simulink model "fft_wideband_real"  (R2012b)
settings: Solver=ode45  StartTime=0.0  StopTime=19999  RelTol=1e-3
undefined symbols (not defined in the file): fft_wideband_real_shift_schedule_user_data_out
libraries: xbsIndex_r4 x8703, xbsReplacements_r4 x36, xps_library x24, dspsigops x16, simulink_xsg_bridge x1
(part 8 of 51)

== system fft_wideband_real/fft_wideband_real/phase_mult/phase12_coeffs ==
  rst : Inport
  Counter : xbsIndex_r4/Counter  cnt_type=Free Running  cnt_to=Inf  operation=Up  start_count=0  cnt_by_val=1  arith_type=Unsigned  n_bits=6  bin_pt=0  load_pin=off  rst=on  en=off  explicit_period=on  period=1  dbl_ovrd=off  use_behavioral_HDL=off  implementation=Fabric  block_type=counter
  Slice : xbsIndex_r4/Slice  nbits=6  boolean_output=off  mode=Upper Bit Location + Width  bit1=0  base1=MSB of Input  bit0=0  base0=LSB of Input  dbl_ovrd=off  block_type=slice
  bram_din_const : xbsIndex_r4/Constant  const=0  gui_display_data_type=Fixed-point  arith_type=Signed (2's comp)  n_bits=18  bin_pt=17  preci_type=Single  exp_width=8  frac_width=24  explicit_period=off  period=1  equ=P=C  opselect=C  inp2=PCIN>>17  opr=+  inp1=P  carry=CIN  dbl_ovrd=off  block_type=constant
  bram_we_const : xbsIndex_r4/Constant  const=0  gui_display_data_type=Fixed-point  arith_type=Boolean  n_bits=16  bin_pt=14  preci_type=Single  exp_width=8  frac_width=24  explicit_period=off  period=1  equ=P=C  opselect=C  inp2=PCIN>>17  opr=+  inp1=P  carry=CIN  dbl_ovrd=off  block_type=constant
  cnt_sign_exta : xbsIndex_r4/Convert  gui_display_data_type=Fixed-point  arith_type=Unsigned  n_bits=10  bin_pt=0  float_type=Single  exp_bits=8  fraction_bits=24  quantization=Truncate  overflow=Wrap  en=off  latency=0  dbl_ovrd=off  pipeline=off  block_type=convert
  cnt_sign_extb : xbsIndex_r4/Convert  gui_display_data_type=Fixed-point  arith_type=Unsigned  n_bits=9  bin_pt=0  float_type=Single  exp_bits=8  fraction_bits=24  quantization=Truncate  overflow=Wrap  en=off  latency=0  dbl_ovrd=off  pipeline=off  block_type=convert
  coeff_mem : xbsIndex_r4/Dual Port RAM  depth=1024  initVector=[1 0.997726440429688 0.99090576171875 0.979568481445312 0.963775634765625 0.943595886230469 0.919113159179688 0.890449523925781 0.85772705078125 0.82110595703125 0.780738830566406 0.73681640625 0.689537048339844 0.639122009277344 0.585800170898438 0.529800415039062 0.471397399902344 0.410842895507812 0.348419189453125 0.284408569335938 0.219100952148438 0.152793884277344 0.0858001708984375 0.0184097290039062 -0.0490646362304688 -0.116317749023438 -0.183036804199219 -0.248924255371094 -0.313682556152344 -0.377006530761719 -0.438613891601562 -0.49822998046875 -0.555572509765625 -0.610382080078125 -0.66241455078125 -0.711433410644531 -0.757209777832031 -0.799537658691406 -0.838226318359375 -0.873092651367188 -0.90399169921875 -0.930763244628906 -0.95330810546875 -0.971504211425781 -0.985275268554688 -0.99456787109375 -0.999320983886719 -0.999526977539062 -0.995185852050781 -0.986305236816406 -0.972938537597656 -0.95513916015625 -0.932991027832031 -0.906593322753906 -0.876068115234375 -0.841552734375 -0.803207397460938 -0.761199951171875 -0.715728759765625 -0.666999816894531 -0.615234375 -0.560661315917969 -0.5035400390625 -0.444122314453125 0 0 0 0 0 0 0 0 0 0 0 0 0 0 0 0 0 0 0 0 0 0 0 0 0 0 0 0 0 0 0 0 0 0 0 0 0 0 0 0 0 0 0 0 0 0 0 0 0 0 0 0 0 0 0 0 0 0 0 0 0 0 0 0 0 0 0 0 0 0 0 0 0 0 0 0 0 0 0 0 0 0 0 0 0 0 0 0 0 0 0 0 0 0 0 0 0 0 0 0 0 0 0 0 0 0 0 0 0 0 0 0 0 0 0 0 0 0 0 0 0 0 0 0 0 0 0 0 0 0 0 0 0 0 0 0 0 0 0 0 0 0 0 0 0 0 0 0 0 0 0 0 0 0 0 0 0 0 0 0 0 0 0 0 0 0 0 0 0 0 0 0 0 0 0 0 0 0 0 0 0 0 0 0 0 0 0 0 0 0 0 0 0 0 0 0 0 0 0 0 0 0 0 0 0 0 0 0 0 0 0 0 0 0 0 0 0 0 0 0 0 0 0 0 0 0 0 0 0 0 0 0 0 0 0 0 0 0 0 0 0 0 0 0 0 0 0 0 0 0 0 0 0 0 0 0 0 0 0 0 0 0 0 0 0 0 0 0 0 0 0 0 0 0 0 0 0 0 0 0 0 0 0 0 0 0 0 0 0 0 0 0 0 0 0 0 0 0 0 0 0 0 0 0 0 0 0 0 0 0 0 0 0 0 0 0 0 0 0 0 0 0 0 0 0 0 0 0 0 0 0 0 0 0 0 0 0 0 0 0 0 0 0 0 0 0 0 0 0 0 0 0 0 0 0 0 0 0 0 0 0 0 0 0 0 0 0 0 0 0 0 0 0 0 0 0 0 0 0 0 0 0 0 0 0 0 0 0 0 0 0 0 0 0 0 0 0 0 0 0 0 0 0 0 0 0 0 0 0 0 0 0 0 0 0 0 0 0 0 0 0 0 0 0 0 0 0 0 0 0 0 0 0 0 0 0 0 0 0 0 0 0 0 0 0 0 0 0 0 -0.06744384765625 -0.13458251953125 -0.201103210449219 -0.266716003417969 -0.331108093261719 -0.393989562988281 -0.455085754394531 -0.51409912109375 -0.570777893066406 -0.624862670898438 -0.676094055175781 -0.724250793457031 -0.76910400390625 -0.810455322265625 -0.848121643066406 -0.881919860839844 -0.911705017089844 -0.937339782714844 -0.958702087402344 -0.975700378417969 -0.988258361816406 -0.996315002441406 -0.999832153320312 -0.998794555664062 -0.993209838867188 -0.983108520507812 -0.968521118164062 -0.949531555175781 -0.92620849609375 -0.898674011230469 -0.867042541503906 -0.831466674804688 -0.792106628417969 -0.749137878417969 -0.702751159667969 -0.653175354003906 -0.600616455078125 -0.545326232910156 -0.487548828125 -0.427558898925781 -0.365615844726562 -0.302009582519531 -0.237022399902344 -0.17095947265625 -0.104118347167969 -0.03680419921875 0.0306777954101562 0.0980148315429688 0.164909362792969 0.231056213378906 0.296150207519531 0.359893798828125 0.4219970703125 0.482185363769531 0.540168762207031 0.595695495605469 0.648513793945312 0.698379516601562 0.74505615234375 0.788345336914062 0.828048706054688 0.863975524902344 0.895965576171875 0 0 0 0 0 0 0 0 0 0 0 0 0 0 0 0 0 0 0 0 0 0 0 0 0 0 0 0 0 0 0 0 0 0 0 0 0 0 0 0 0 0 0 0 0 0 0 0 0 0 0 0 0 0 0 0 0 0 0 0 0 0 0 0 0 0 0 0 0 0 0 0 0 0 0 0 0 0 0 0 0 0 0 0 0 0 0 0 0 0 0 0 0 0 0 0 0 0 0 0 0 0 0 0 0 0 0 0 0 0 0 0 0 0 0 0 0 0 0 0 0 0 0 0 0 0 0 0 0 0 0 0 0 0 0 0 0 0 0 0 0 0 0 0 0 0 0 0 0 0 0 0 0 0 0 0 0 0 0 0 0 0 0 0 0 0 0 0 0 0 0 0 0 0 0 0 0 0 0 0 0 0 0 0 0 0 0 0 0 0 0 0 0 0 0 0 0 0 0 0 0 0 0 0 0 0 0 0 0 0 0 0 0 0 0 0 0 0 0 0 0 0 0 0 0 0 0 0 0 0 0 0 0 0 0 0 0 0 0 0 0 0 0 0 0 0 0 0 0 0 0 0 0 0 0 0 0 0 0 0 0 0 0 0 0 0 0 0 0 0 0 0 0 0 0 0 0 0 0 0 0 0 0 0 0 0 0 0 0 0 0 0 0 0 0 0 0 0 0 0 0 0 0 0 0 0 0 0 0 0 0 0 0 0 0 0 0 0 0 0 0 0 0 0 0 0 0 0 0 0 0 0 0 0 0 0 0 0 0 0 0 0 0 0 0 0 0 0 0 0 0 0 0 0 0 0 0 0 0 0 0 0 0 0 0 0 0 0 0 0 0 0 0 0 0 0 0 0 0 0 0 0 0 0 0 0 0 0 0 0 0 0 0 0 0 0 0 0 0 0 0 0 0 0 0 0 0 0 0 0 0 0 0 0 0 0 0 0 0 0 0 0 0 0 0 0 0 0 0 0 0 0 0 0 0 0 0 0 0 0 0 0 0 0 0 0 0 0]  distributed_mem=Block RAM  init_a=0  init_b=0  rst_a=off  rst_b=off  en_a=off  en_b=off  latency=2  write_mode_A=Read After Write  write_mode_B=Read After Write  dbl_ovrd=off  optimize=Area  use_rpm=on  block_type=dpram
  counter_b_concat : xbsIndex_r4/Concat  num_inputs=2  dbl_ovrd=off  block_type=concat
  counter_b_pad : xbsIndex_r4/Constant  const=1  gui_display_data_type=Fixed-point  arith_type=Unsigned  n_bits=1  bin_pt=0  preci_type=Single  exp_width=8  frac_width=24  explicit_period=off  period=1  equ=P=C  opselect=C  inp2=PCIN>>17  opr=+  inp1=P  carry=CIN  dbl_ovrd=off  block_type=constant
  ri_to_c : Subsystem
  w : Outport
  wires:
  Slice/1 -> cnt_sign_extb/1, cnt_sign_exta/1
  bram_din_const/1 -> coeff_mem/5, coeff_mem/2
  bram_we_const/1 -> coeff_mem/6, coeff_mem/3
  ri_to_c/1(c) -> w/1
  coeff_mem/2 -> ri_to_c/2(im)
  coeff_mem/1 -> ri_to_c/1(re)
  counter_b_concat/1 -> coeff_mem/4
  cnt_sign_exta/1 -> coeff_mem/1
  cnt_sign_extb/1 -> counter_b_concat/2
  counter_b_pad/1 -> counter_b_concat/1
  Counter/1 -> Slice/1
  rst/1 -> Counter/1

== system fft_wideband_real/fft_wideband_real/phase_mult/phase13_coeffs ==
  rst : Inport
  Counter : xbsIndex_r4/Counter  cnt_type=Free Running  cnt_to=Inf  operation=Up  start_count=0  cnt_by_val=1  arith_type=Unsigned  n_bits=6  bin_pt=0  load_pin=off  rst=on  en=off  explicit_period=on  period=1  dbl_ovrd=off  use_behavioral_HDL=off  implementation=Fabric  block_type=counter
  Slice : xbsIndex_r4/Slice  nbits=6  boolean_output=off  mode=Upper Bit Location + Width  bit1=0  base1=MSB of Input  bit0=0  base0=LSB of Input  dbl_ovrd=off  block_type=slice
  bram_din_const : xbsIndex_r4/Constant  const=0  gui_display_data_type=Fixed-point  arith_type=Signed (2's comp)  n_bits=18  bin_pt=17  preci_type=Single  exp_width=8  frac_width=24  explicit_period=off  period=1  equ=P=C  opselect=C  inp2=PCIN>>17  opr=+  inp1=P  carry=CIN  dbl_ovrd=off  block_type=constant
  bram_we_const : xbsIndex_r4/Constant  const=0  gui_display_data_type=Fixed-point  arith_type=Boolean  n_bits=16  bin_pt=14  preci_type=Single  exp_width=8  frac_width=24  explicit_period=off  period=1  equ=P=C  opselect=C  inp2=PCIN>>17  opr=+  inp1=P  carry=CIN  dbl_ovrd=off  block_type=constant
  cnt_sign_exta : xbsIndex_r4/Convert  gui_display_data_type=Fixed-point  arith_type=Unsigned  n_bits=10  bin_pt=0  float_type=Single  exp_bits=8  fraction_bits=24  quantization=Truncate  overflow=Wrap  en=off  latency=0  dbl_ovrd=off  pipeline=off  block_type=convert
  cnt_sign_extb : xbsIndex_r4/Convert  gui_display_data_type=Fixed-point  arith_type=Unsigned  n_bits=9  bin_pt=0  float_type=Single  exp_bits=8  fraction_bits=24  quantization=Truncate  overflow=Wrap  en=off  latency=0  dbl_ovrd=off  pipeline=off  block_type=convert
  coeff_mem : xbsIndex_r4/Dual Port RAM  depth=1024  initVector=[1 0.997291564941406 0.989173889160156 0.975700378417969 0.956939697265625 0.932991027832031 0.90399169921875 0.870086669921875 0.831466674804688 0.788345336914062 0.740951538085938 0.689537048339844 0.634391784667969 0.5758056640625 0.51409912109375 0.449607849121094 0.382682800292969 0.313682556152344 0.24298095703125 0.17095947265625 0.0980148315429688 0.0245437622070312 -0.0490646362304688 -0.122413635253906 -0.195091247558594 -0.266716003417969 -0.336891174316406 -0.405242919921875 -0.471397399902344 -0.534996032714844 -0.595695495605469 -0.653175354003906 -0.707107543945312 -0.757209777832031 -0.803207397460938 -0.844856262207031 -0.881919860839844 -0.914207458496094 -0.941543579101562 -0.963775634765625 -0.980781555175781 -0.992477416992188 -0.998794555664062 -0.999702453613281 -0.995185852050781 -0.985275268554688 -0.97003173828125 -0.949531555175781 -0.923881530761719 -0.893226623535156 -0.85772705078125 -0.817581176757812 -0.77301025390625 -0.724250793457031 -0.671562194824219 -0.615234375 -0.555572509765625 -0.492897033691406 -0.427558898925781 -0.359893798828125 -0.290283203125 -0.219100952148438 -0.146728515625 -0.0735626220703125 0 0 0 0 0 0 0 0 0 0 0 0 0 0 0 0 0 0 0 0 0 0 0 0 0 0 0 0 0 0 0 0 0 0 0 0 0 0 0 0 0 0 0 0 0 0 0 0 0 0 0 0 0 0 0 0 0 0 0 0 0 0 0 0 0 0 0 0 0 0 0 0 0 0 0 0 0 0 0 0 0 0 0 0 0 0 0 0 0 0 0 0 0 0 0 0 0 0 0 0 0 0 0 0 0 0 0 0 0 0 0 0 0 0 0 0 0 0 0 0 0 0 0 0 0 0 0 0 0 0 0 0 0 0 0 0 0 0 0 0 0 0 0 0 0 0 0 0 0 0 0 0 0 0 0 0 0 0 0 0 0 0 0 0 0 0 0 0 0 0 0 0 0 0 0 0 0 0 0 0 0 0 0 0 0 0 0 0 0 0 0 0 0 0 0 0 0 0 0 0 0 0 0 0 0 0 0 0 0 0 0 0 0 0 0 0 0 0 0 0 0 0 0 0 0 0 0 0 0 0 0 0 0 0 0 0 0 0 0 0 0 0 0 0 0 0 0 0 0 0 0 0 0 0 0 0 0 0 0 0 0 0 0 0 0 0 0 0 0 0 0 0 0 0 0 0 0 0 0 0 0 0 0 0 0 0 0 0 0 0 0 0 0 0 0 0 0 0 0 0 0 0 0 0 0 0 0 0 0 0 0 0 0 0 0 0 0 0 0 0 0 0 0 0 0 0 0 0 0 0 0 0 0 0 0 0 0 0 0 0 0 0 0 0 0 0 0 0 0 0 0 0 0 0 0 0 0 0 0 0 0 0 0 0 0 0 0 0 0 0 0 0 0 0 0 0 0 0 0 0 0 0 0 0 0 0 0 0 0 0 0 0 0 0 0 0 0 0 0 0 0 0 0 0 0 0 0 0 0 0 0 0 0 0 0 0 0 0 0 0 0 0 0 0 0 0 0 0 0 0 0 0 0 0 0 0 0 0 0 0 0 0 0 0 0 0 0 0 0 -0.0735626220703125 -0.146728515625 -0.219100952148438 -0.290283203125 -0.359893798828125 -0.427558898925781 -0.492897033691406 -0.555572509765625 -0.615234375 -0.671562194824219 -0.724250793457031 -0.77301025390625 -0.817581176757812 -0.85772705078125 -0.893226623535156 -0.923881530761719 -0.949531555175781 -0.97003173828125 -0.985275268554688 -0.995185852050781 -0.999702453613281 -0.998794555664062 -0.992477416992188 -0.980781555175781 -0.963775634765625 -0.941543579101562 -0.914207458496094 -0.881919860839844 -0.844856262207031 -0.803207397460938 -0.757209777832031 -0.707107543945312 -0.653175354003906 -0.595695495605469 -0.534996032714844 -0.471397399902344 -0.405242919921875 -0.336891174316406 -0.266716003417969 -0.195091247558594 -0.122413635253906 -0.0490646362304688 0.0245437622070312 0.0980148315429688 0.17095947265625 0.24298095703125 0.313682556152344 0.382682800292969 0.449607849121094 0.51409912109375 0.5758056640625 0.634391784667969 0.689537048339844 0.740951538085938 0.788345336914062 0.831466674804688 0.870086669921875 0.90399169921875 0.932991027832031 0.956939697265625 0.975700378417969 0.989173889160156 0.997291564941406 0 0 0 0 0 0 0 0 0 0 0 0 0 0 0 0 0 0 0 0 0 0 0 0 0 0 0 0 0 0 0 0 0 0 0 0 0 0 0 0 0 0 0 0 0 0 0 0 0 0 0 0 0 0 0 0 0 0 0 0 0 0 0 0 0 0 0 0 0 0 0 0 0 0 0 0 0 0 0 0 0 0 0 0 0 0 0 0 0 0 0 0 0 0 0 0 0 0 0 0 0 0 0 0 0 0 0 0 0 0 0 0 0 0 0 0 0 0 0 0 0 0 0 0 0 0 0 0 0 0 0 0 0 0 0 0 0 0 0 0 0 0 0 0 0 0 0 0 0 0 0 0 0 0 0 0 0 0 0 0 0 0 0 0 0 0 0 0 0 0 0 0 0 0 0 0 0 0 0 0 0 0 0 0 0 0 0 0 0 0 0 0 0 0 0 0 0 0 0 0 0 0 0 0 0 0 0 0 0 0 0 0 0 0 0 0 0 0 0 0 0 0 0 0 0 0 0 0 0 0 0 0 0 0 0 0 0 0 0 0 0 0 0 0 0 0 0 0 0 0 0 0 0 0 0 0 0 0 0 0 0 0 0 0 0 0 0 0 0 0 0 0 0 0 0 0 0 0 0 0 0 0 0 0 0 0 0 0 0 0 0 0 0 0 0 0 0 0 0 0 0 0 0 0 0 0 0 0 0 0 0 0 0 0 0 0 0 0 0 0 0 0 0 0 0 0 0 0 0 0 0 0 0 0 0 0 0 0 0 0 0 0 0 0 0 0 0 0 0 0 0 0 0 0 0 0 0 0 0 0 0 0 0 0 0 0 0 0 0 0 0 0 0 0 0 0 0 0 0 0 0 0 0 0 0 0 0 0 0 0 0 0 0 0 0 0 0 0 0 0 0 0 0 0 0 0 0 0 0 0 0 0 0 0 0 0 0 0 0 0 0 0 0 0 0 0 0 0 0 0 0 0 0 0 0 0 0 0 0 0 0 0 0 0 0 0 0 0]  distributed_mem=Block RAM  init_a=0  init_b=0  rst_a=off  rst_b=off  en_a=off  en_b=off  latency=2  write_mode_A=Read After Write  write_mode_B=Read After Write  dbl_ovrd=off  optimize=Area  use_rpm=on  block_type=dpram
  counter_b_concat : xbsIndex_r4/Concat  num_inputs=2  dbl_ovrd=off  block_type=concat
  counter_b_pad : xbsIndex_r4/Constant  const=1  gui_display_data_type=Fixed-point  arith_type=Unsigned  n_bits=1  bin_pt=0  preci_type=Single  exp_width=8  frac_width=24  explicit_period=off  period=1  equ=P=C  opselect=C  inp2=PCIN>>17  opr=+  inp1=P  carry=CIN  dbl_ovrd=off  block_type=constant
  ri_to_c : Subsystem
  w : Outport
  wires:
  Slice/1 -> cnt_sign_extb/1, cnt_sign_exta/1
  bram_din_const/1 -> coeff_mem/5, coeff_mem/2
  bram_we_const/1 -> coeff_mem/6, coeff_mem/3
  ri_to_c/1(c) -> w/1
  coeff_mem/2 -> ri_to_c/2(im)
  coeff_mem/1 -> ri_to_c/1(re)
  counter_b_concat/1 -> coeff_mem/4
  cnt_sign_exta/1 -> coeff_mem/1
  cnt_sign_extb/1 -> counter_b_concat/2
  counter_b_pad/1 -> counter_b_concat/1
  Counter/1 -> Slice/1
  rst/1 -> Counter/1

== system fft_wideband_real/fft_wideband_real/phase_mult/phase14_coeffs ==
  rst : Inport
  Counter : xbsIndex_r4/Counter  cnt_type=Free Running  cnt_to=Inf  operation=Up  start_count=0  cnt_by_val=1  arith_type=Unsigned  n_bits=6  bin_pt=0  load_pin=off  rst=on  en=off  explicit_period=on  period=1  dbl_ovrd=off  use_behavioral_HDL=off  implementation=Fabric  block_type=counter
  Slice : xbsIndex_r4/Slice  nbits=6  boolean_output=off  mode=Upper Bit Location + Width  bit1=0  base1=MSB of Input  bit0=0  base0=LSB of Input  dbl_ovrd=off  block_type=slice
  bram_din_const : xbsIndex_r4/Constant  const=0  gui_display_data_type=Fixed-point  arith_type=Signed (2's comp)  n_bits=18  bin_pt=17  preci_type=Single  exp_width=8  frac_width=24  explicit_period=off  period=1  equ=P=C  opselect=C  inp2=PCIN>>17  opr=+  inp1=P  carry=CIN  dbl_ovrd=off  block_type=constant
  bram_we_const : xbsIndex_r4/Constant  const=0  gui_display_data_type=Fixed-point  arith_type=Boolean  n_bits=16  bin_pt=14  preci_type=Single  exp_width=8  frac_width=24  explicit_period=off  period=1  equ=P=C  opselect=C  inp2=PCIN>>17  opr=+  inp1=P  carry=CIN  dbl_ovrd=off  block_type=constant
  cnt_sign_exta : xbsIndex_r4/Convert  gui_display_data_type=Fixed-point  arith_type=Unsigned  n_bits=10  bin_pt=0  float_type=Single  exp_bits=8  fraction_bits=24  quantization=Truncate  overflow=Wrap  en=off  latency=0  dbl_ovrd=off  pipeline=off  block_type=convert
  cnt_sign_extb : xbsIndex_r4/Convert  gui_display_data_type=Fixed-point  arith_type=Unsigned  n_bits=9  bin_pt=0  float_type=Single  exp_bits=8  fraction_bits=24  quantization=Truncate  overflow=Wrap  en=off  latency=0  dbl_ovrd=off  pipeline=off  block_type=convert
  coeff_mem : xbsIndex_r4/Dual Port RAM  depth=1024  initVector=[1 0.996818542480469 0.9873046875 0.971504211425781 0.949531555175781 0.921516418457031 0.887641906738281 0.848121643066406 0.803207397460938 0.753189086914062 0.698379516601562 0.639122009277344 0.5758056640625 0.508827209472656 0.438613891601562 0.365615844726562 0.290283203125 0.213111877441406 0.13458251953125 0.0551986694335938 -0.0245437622070312 -0.104118347167969 -0.183036804199219 -0.260795593261719 -0.336891174316406 -0.410842895507812 -0.482185363769531 -0.550460815429688 -0.615234375 -0.676094055175781 -0.732650756835938 -0.784553527832031 -0.831466674804688 -0.873092651367188 -0.909164428710938 -0.939460754394531 -0.963775634765625 -0.981964111328125 -0.993904113769531 -0.999526977539062 -0.998794555664062 -0.991706848144531 -0.978317260742188 -0.958702087402344 -0.932991027832031 -0.901351928710938 -0.863975524902344 -0.82110595703125 -0.77301025390625 -0.720001220703125 -0.66241455078125 -0.600616455078125 -0.534996032714844 -0.465972900390625 -0.393989562988281 -0.319503784179688 -0.24298095703125 -0.164909362792969 -0.0858001708984375 -0.006134033203125 0.0735626220703125 0.152793884277344 0.231056213378906 0.307846069335938 0 0 0 0 0 0 0 0 0 0 0 0 0 0 0 0 0 0 0 0 0 0 0 0 0 0 0 0 0 0 0 0 0 0 0 0 0 0 0 0 0 0 0 0 0 0 0 0 0 0 0 0 0 0 0 0 0 0 0 0 0 0 0 0 0 0 0 0 0 0 0 0 0 0 0 0 0 0 0 0 0 0 0 0 0 0 0 0 0 0 0 0 0 0 0 0 0 0 0 0 0 0 0 0 0 0 0 0 0 0 0 0 0 0 0 0 0 0 0 0 0 0 0 0 0 0 0 0 0 0 0 0 0 0 0 0 0 0 0 0 0 0 0 0 0 0 0 0 0 0 0 0 0 0 0 0 0 0 0 0 0 0 0 0 0 0 0 0 0 0 0 0 0 0 0 0 0 0 0 0 0 0 0 0 0 0 0 0 0 0 0 0 0 0 0 0 0 0 0 0 0 0 0 0 0 0 0 0 0 0 0 0 0 0 0 0 0 0 0 0 0 0 0 0 0 0 0 0 0 0 0 0 0 0 0 0 0 0 0 0 0 0 0 0 0 0 0 0 0 0 0 0 0 0 0 0 0 0 0 0 0 0 0 0 0 0 0 0 0 0 0 0 0 0 0 0 0 0 0 0 0 0 0 0 0 0 0 0 0 0 0 0 0 0 0 0 0 0 0 0 0 0 0 0 0 0 0 0 0 0 0 0 0 0 0 0 0 0 0 0 0 0 0 0 0 0 0 0 0 0 0 0 0 0 0 0 0 0 0 0 0 0 0 0 0 0 0 0 0 0 0 0 0 0 0 0 0 0 0 0 0 0 0 0 0 0 0 0 0 0 0 0 0 0 0 0 0 0 0 0 0 0 0 0 0 0 0 0 0 0 0 0 0 0 0 0 0 0 0 0 0 0 0 0 0 0 0 0 0 0 0 0 0 0 0 0 0 0 0 0 0 0 0 0 0 0 0 0 0 0 0 0 0 0 0 0 0 0 0 0 0 0 0 0 0 0 0 0 0 -0.079681396484375 -0.158859252929688 -0.237022399902344 -0.313682556152344 -0.388343811035156 -0.460540771484375 -0.529800415039062 -0.595695495605469 -0.657806396484375 -0.715728759765625 -0.76910400390625 -0.817581176757812 -0.860870361328125 -0.898674011230469 -0.930763244628906 -0.956939697265625 -0.977027893066406 -0.99090576171875 -0.99847412109375 -0.999702453613281 -0.99456787109375 -0.983108520507812 -0.96539306640625 -0.941543579101562 -0.911705017089844 -0.876068115234375 -0.834861755371094 -0.788345336914062 -0.73681640625 -0.68060302734375 -0.62005615234375 -0.555572509765625 -0.487548828125 -0.416427612304688 -0.342658996582031 -0.266716003417969 -0.189071655273438 -0.110221862792969 -0.0306777954101562 0.0490646362304688 0.128501892089844 0.207115173339844 0.284408569335938 0.359893798828125 0.433090209960938 0.5035400390625 0.570777893066406 0.634391784667969 0.6939697265625 0.749137878417969 0.799537658691406 0.844856262207031 0.884796142578125 0.919113159179688 0.947586059570312 0.97003173828125 0.986305236816406 0.996315002441406 0.999984741210938 0.997291564941406 0.988258361816406 0.972938537597656 0.951431274414062 0 0 0 0 0 0 0 0 0 0 0 0 0 0 0 0 0 0 0 0 0 0 0 0 0 0 0 0 0 0 0 0 0 0 0 0 0 0 0 0 0 0 0 0 0 0 0 0 0 0 0 0 0 0 0 0 0 0 0 0 0 0 0 0 0 0 0 0 0 0 0 0 0 0 0 0 0 0 0 0 0 0 0 0 0 0 0 0 0 0 0 0 0 0 0 0 0 0 0 0 0 0 0 0 0 0 0 0 0 0 0 0 0 0 0 0 0 0 0 0 0 0 0 0 0 0 0 0 0 0 0 0 0 0 0 0 0 0 0 0 0 0 0 0 0 0 0 0 0 0 0 0 0 0 0 0 0 0 0 0 0 0 0 0 0 0 0 0 0 0 0 0 0 0 0 0 0 0 0 0 0 0 0 0 0 0 0 0 0 0 0 0 0 0 0 0 0 0 0 0 0 0 0 0 0 0 0 0 0 0 0 0 0 0 0 0 0 0 0 0 0 0 0 0 0 0 0 0 0 0 0 0 0 0 0 0 0 0 0 0 0 0 0 0 0 0 0 0 0 0 0 0 0 0 0 0 0 0 0 0 0 0 0 0 0 0 0 0 0 0 0 0 0 0 0 0 0 0 0 0 0 0 0 0 0 0 0 0 0 0 0 0 0 0 0 0 0 0 0 0 0 0 0 0 0 0 0 0 0 0 0 0 0 0 0 0 0 0 0 0 0 0 0 0 0 0 0 0 0 0 0 0 0 0 0 0 0 0 0 0 0 0 0 0 0 0 0 0 0 0 0 0 0 0 0 0 0 0 0 0 0 0 0 0 0 0 0 0 0 0 0 0 0 0 0 0 0 0 0 0 0 0 0 0 0 0 0 0 0 0 0 0 0 0 0 0 0 0 0 0 0 0 0 0 0 0 0 0 0 0 0 0 0 0 0 0 0 0 0 0 0 0 0 0 0 0 0 0 0 0 0 0 0 0 0 0 0 0 0 0 0 0 0 0 0 0 0 0]  distributed_mem=Block RAM  init_a=0  init_b=0  rst_a=off  rst_b=off  en_a=off  en_b=off  latency=2  write_mode_A=Read After Write  write_mode_B=Read After Write  dbl_ovrd=off  optimize=Area  use_rpm=on  block_type=dpram
  counter_b_concat : xbsIndex_r4/Concat  num_inputs=2  dbl_ovrd=off  block_type=concat
  counter_b_pad : xbsIndex_r4/Constant  const=1  gui_display_data_type=Fixed-point  arith_type=Unsigned  n_bits=1  bin_pt=0  preci_type=Single  exp_width=8  frac_width=24  explicit_period=off  period=1  equ=P=C  opselect=C  inp2=PCIN>>17  opr=+  inp1=P  carry=CIN  dbl_ovrd=off  block_type=constant
  ri_to_c : Subsystem
  w : Outport
  wires:
  Slice/1 -> cnt_sign_extb/1, cnt_sign_exta/1
  bram_din_const/1 -> coeff_mem/5, coeff_mem/2
  bram_we_const/1 -> coeff_mem/6, coeff_mem/3
  ri_to_c/1(c) -> w/1
  coeff_mem/2 -> ri_to_c/2(im)
  coeff_mem/1 -> ri_to_c/1(re)
  counter_b_concat/1 -> coeff_mem/4
  cnt_sign_exta/1 -> coeff_mem/1
  cnt_sign_extb/1 -> counter_b_concat/2
  counter_b_pad/1 -> counter_b_concat/1
  Counter/1 -> Slice/1
  rst/1 -> Counter/1

== system fft_wideband_real/fft_wideband_real/phase_mult/phase15_coeffs ==
  rst : Inport
  Counter : xbsIndex_r4/Counter  cnt_type=Free Running  cnt_to=Inf  operation=Up  start_count=0  cnt_by_val=1  arith_type=Unsigned  n_bits=6  bin_pt=0  load_pin=off  rst=on  en=off  explicit_period=on  period=1  dbl_ovrd=off  use_behavioral_HDL=off  implementation=Fabric  block_type=counter
  Slice : xbsIndex_r4/Slice  nbits=6  boolean_output=off  mode=Upper Bit Location + Width  bit1=0  base1=MSB of Input  bit0=0  base0=LSB of Input  dbl_ovrd=off  block_type=slice
  bram_din_const : xbsIndex_r4/Constant  const=0  gui_display_data_type=Fixed-point  arith_type=Signed (2's comp)  n_bits=18  bin_pt=17  preci_type=Single  exp_width=8  frac_width=24  explicit_period=off  period=1  equ=P=C  opselect=C  inp2=PCIN>>17  opr=+  inp1=P  carry=CIN  dbl_ovrd=off  block_type=constant
  bram_we_const : xbsIndex_r4/Constant  const=0  gui_display_data_type=Fixed-point  arith_type=Boolean  n_bits=16  bin_pt=14  preci_type=Single  exp_width=8  frac_width=24  explicit_period=off  period=1  equ=P=C  opselect=C  inp2=PCIN>>17  opr=+  inp1=P  carry=CIN  dbl_ovrd=off  block_type=constant
  cnt_sign_exta : xbsIndex_r4/Convert  gui_display_data_type=Fixed-point  arith_type=Unsigned  n_bits=10  bin_pt=0  float_type=Single  exp_bits=8  fraction_bits=24  quantization=Truncate  overflow=Wrap  en=off  latency=0  dbl_ovrd=off  pipeline=off  block_type=convert
  cnt_sign_extb : xbsIndex_r4/Convert  gui_display_data_type=Fixed-point  arith_type=Unsigned  n_bits=9  bin_pt=0  float_type=Single  exp_bits=8  fraction_bits=24  quantization=Truncate  overflow=Wrap  en=off  latency=0  dbl_ovrd=off  pipeline=off  block_type=convert
  coeff_mem : xbsIndex_r4/Dual Port RAM  depth=1024  initVector=[1 0.996315002441406 0.985275268554688 0.96697998046875 0.941543579101562 0.909164428710938 0.870086669921875 0.824592590332031 0.77301025390625 0.715728759765625 0.653175354003906 0.585800170898438 0.51409912109375 0.438613891601562 0.359893798828125 0.278518676757812 0.195091247558594 0.110221862792969 0.0245437622070312 -0.0613174438476562 -0.146728515625 -0.231056213378906 -0.313682556152344 -0.393989562988281 -0.471397399902344 -0.545326232910156 -0.615234375 -0.68060302734375 -0.740951538085938 -0.79583740234375 -0.844856262207031 -0.887641906738281 -0.923881530761719 -0.95330810546875 -0.975700378417969 -0.99090576171875 -0.998794555664062 -0.999320983886719 -0.992477416992188 -0.978317260742188 -0.956939697265625 -0.928504943847656 -0.893226623535156 -0.851356506347656 -0.803207397460938 -0.749137878417969 -0.689537048339844 -0.624862670898438 -0.555572509765625 -0.482185363769531 -0.405242919921875 -0.325309753417969 -0.24298095703125 -0.158859252929688 -0.0735626220703125 0.01226806640625 0.0980148315429688 0.183036804199219 0.266716003417969 0.348419189453125 0.427558898925781 0.5035400390625 0.5758056640625 0.643829345703125 0 0 0 0 0 0 0 0 0 0 0 0 0 0 0 0 0 0 0 0 0 0 0 0 0 0 0 0 0 0 0 0 0 0 0 0 0 0 0 0 0 0 0 0 0 0 0 0 0 0 0 0 0 0 0 0 0 0 0 0 0 0 0 0 0 0 0 0 0 0 0 0 0 0 0 0 0 0 0 0 0 0 0 0 0 0 0 0 0 0 0 0 0 0 0 0 0 0 0 0 0 0 0 0 0 0 0 0 0 0 0 0 0 0 0 0 0 0 0 0 0 0 0 0 0 0 0 0 0 0 0 0 0 0 0 0 0 0 0 0 0 0 0 0 0 0 0 0 0 0 0 0 0 0 0 0 0 0 0 0 0 0 0 0 0 0 0 0 0 0 0 0 0 0 0 0 0 0 0 0 0 0 0 0 0 0 0 0 0 0 0 0 0 0 0 0 0 0 0 0 0 0 0 0 0 0 0 0 0 0 0 0 0 0 0 0 0 0 0 0 0 0 0 0 0 0 0 0 0 0 0 0 0 0 0 0 0 0 0 0 0 0 0 0 0 0 0 0 0 0 0 0 0 0 0 0 0 0 0 0 0 0 0 0 0 0 0 0 0 0 0 0 0 0 0 0 0 0 0 0 0 0 0 0 0 0 0 0 0 0 0 0 0 0 0 0 0 0 0 0 0 0 0 0 0 0 0 0 0 0 0 0 0 0 0 0 0 0 0 0 0 0 0 0 0 0 0 0 0 0 0 0 0 0 0 0 0 0 0 0 0 0 0 0 0 0 0 0 0 0 0 0 0 0 0 0 0 0 0 0 0 0 0 0 0 0 0 0 0 0 0 0 0 0 0 0 0 0 0 0 0 0 0 0 0 0 0 0 0 0 0 0 0 0 0 0 0 0 0 0 0 0 0 0 0 0 0 0 0 0 0 0 0 0 0 0 0 0 0 0 0 0 0 0 0 0 0 0 0 0 0 0 0 0 0 0 0 0 0 0 0 0 0 0 0 0 0 0 0 -0.0858001708984375 -0.17095947265625 -0.254867553710938 -0.336891174316406 -0.416427612304688 -0.492897033691406 -0.56573486328125 -0.634391784667969 -0.698379516601562 -0.757209777832031 -0.810455322265625 -0.85772705078125 -0.898674011230469 -0.932991027832031 -0.960433959960938 -0.980781555175781 -0.993904113769531 -0.999702453613281 -0.998115539550781 -0.989173889160156 -0.972938537597656 -0.949531555175781 -0.919113159179688 -0.881919860839844 -0.838226318359375 -0.788345336914062 -0.732650756835938 -0.671562194824219 -0.605514526367188 -0.534996032714844 -0.460540771484375 -0.382682800292969 -0.302009582519531 -0.219100952148438 -0.13458251953125 -0.0490646362304688 0.03680419921875 0.122413635253906 0.207115173339844 0.290283203125 0.371315002441406 0.449607849121094 0.524589538574219 0.595695495605469 0.66241455078125 0.724250793457031 0.780738830566406 0.831466674804688 0.876068115234375 0.914207458496094 0.945610046386719 0.97003173828125 0.9873046875 0.997291564941406 0.999923706054688 0.995185852050781 0.983108520507812 0.963775634765625 0.937339782714844 0.90399169921875 0.863975524902344 0.817581176757812 0.765167236328125 0 0 0 0 0 0 0 0 0 0 0 0 0 0 0 0 0 0 0 0 0 0 0 0 0 0 0 0 0 0 0 0 0 0 0 0 0 0 0 0 0 0 0 0 0 0 0 0 0 0 0 0 0 0 0 0 0 0 0 0 0 0 0 0 0 0 0 0 0 0 0 0 0 0 0 0 0 0 0 0 0 0 0 0 0 0 0 0 0 0 0 0 0 0 0 0 0 0 0 0 0 0 0 0 0 0 0 0 0 0 0 0 0 0 0 0 0 0 0 0 0 0 0 0 0 0 0 0 0 0 0 0 0 0 0 0 0 0 0 0 0 0 0 0 0 0 0 0 0 0 0 0 0 0 0 0 0 0 0 0 0 0 0 0 0 0 0 0 0 0 0 0 0 0 0 0 0 0 0 0 0 0 0 0 0 0 0 0 0 0 0 0 0 0 0 0 0 0 0 0 0 0 0 0 0 0 0 0 0 0 0 0 0 0 0 0 0 0 0 0 0 0 0 0 0 0 0 0 0 0 0 0 0 0 0 0 0 0 0 0 0 0 0 0 0 0 0 0 0 0 0 0 0 0 0 0 0 0 0 0 0 0 0 0 0 0 0 0 0 0 0 0 0 0 0 0 0 0 0 0 0 0 0 0 0 0 0 0 0 0 0 0 0 0 0 0 0 0 0 0 0 0 0 0 0 0 0 0 0 0 0 0 0 0 0 0 0 0 0 0 0 0 0 0 0 0 0 0 0 0 0 0 0 0 0 0 0 0 0 0 0 0 0 0 0 0 0 0 0 0 0 0 0 0 0 0 0 0 0 0 0 0 0 0 0 0 0 0 0 0 0 0 0 0 0 0 0 0 0 0 0 0 0 0 0 0 0 0 0 0 0 0 0 0 0 0 0 0 0 0 0 0 0 0 0 0 0 0 0 0 0 0 0 0 0 0 0 0 0 0 0 0 0 0 0 0 0 0 0 0 0 0 0 0 0 0 0 0 0 0 0 0 0 0 0 0 0 0]  distributed_mem=Block RAM  init_a=0  init_b=0  rst_a=off  rst_b=off  en_a=off  en_b=off  latency=2  write_mode_A=Read After Write  write_mode_B=Read After Write  dbl_ovrd=off  optimize=Area  use_rpm=on  block_type=dpram
  counter_b_concat : xbsIndex_r4/Concat  num_inputs=2  dbl_ovrd=off  block_type=concat
  counter_b_pad : xbsIndex_r4/Constant  const=1  gui_display_data_type=Fixed-point  arith_type=Unsigned  n_bits=1  bin_pt=0  preci_type=Single  exp_width=8  frac_width=24  explicit_period=off  period=1  equ=P=C  opselect=C  inp2=PCIN>>17  opr=+  inp1=P  carry=CIN  dbl_ovrd=off  block_type=constant
  ri_to_c : Subsystem
  w : Outport
  wires:
  Slice/1 -> cnt_sign_extb/1, cnt_sign_exta/1
  bram_din_const/1 -> coeff_mem/5, coeff_mem/2
  bram_we_const/1 -> coeff_mem/6, coeff_mem/3
  ri_to_c/1(c) -> w/1
  coeff_mem/2 -> ri_to_c/2(im)
  coeff_mem/1 -> ri_to_c/1(re)
  counter_b_concat/1 -> coeff_mem/4
  cnt_sign_exta/1 -> coeff_mem/1
  cnt_sign_extb/1 -> counter_b_concat/2
  counter_b_pad/1 -> counter_b_concat/1
  Counter/1 -> Slice/1
  rst/1 -> Counter/1

== system fft_wideband_real/fft_wideband_real/phase_mult/phase16_coeffs ==
  rst : Inport
  Counter : xbsIndex_r4/Counter  cnt_type=Free Running  cnt_to=Inf  operation=Up  start_count=0  cnt_by_val=1  arith_type=Unsigned  n_bits=6  bin_pt=0  load_pin=off  rst=on  en=off  explicit_period=on  period=1  dbl_ovrd=off  use_behavioral_HDL=off  implementation=Fabric  block_type=counter
  Slice : xbsIndex_r4/Slice  nbits=6  boolean_output=off  mode=Upper Bit Location + Width  bit1=0  base1=MSB of Input  bit0=0  base0=LSB of Input  dbl_ovrd=off  block_type=slice
  bram_din_const : xbsIndex_r4/Constant  const=0  gui_display_data_type=Fixed-point  arith_type=Signed (2's comp)  n_bits=18  bin_pt=17  preci_type=Single  exp_width=8  frac_width=24  explicit_period=off  period=1  equ=P=C  opselect=C  inp2=PCIN>>17  opr=+  inp1=P  carry=CIN  dbl_ovrd=off  block_type=constant
  bram_we_const : xbsIndex_r4/Constant  const=0  gui_display_data_type=Fixed-point  arith_type=Boolean  n_bits=16  bin_pt=14  preci_type=Single  exp_width=8  frac_width=24  explicit_period=off  period=1  equ=P=C  opselect=C  inp2=PCIN>>17  opr=+  inp1=P  carry=CIN  dbl_ovrd=off  block_type=constant
  cnt_sign_exta : xbsIndex_r4/Convert  gui_display_data_type=Fixed-point  arith_type=Unsigned  n_bits=10  bin_pt=0  float_type=Single  exp_bits=8  fraction_bits=24  quantization=Truncate  overflow=Wrap  en=off  latency=0  dbl_ovrd=off  pipeline=off  block_type=convert
  cnt_sign_extb : xbsIndex_r4/Convert  gui_display_data_type=Fixed-point  arith_type=Unsigned  n_bits=9  bin_pt=0  float_type=Single  exp_bits=8  fraction_bits=24  quantization=Truncate  overflow=Wrap  en=off  latency=0  dbl_ovrd=off  pipeline=off  block_type=convert
  coeff_mem : xbsIndex_r4/Dual Port RAM  depth=1024  initVector=[1 0.995765686035156 0.983108520507812 0.962120056152344 0.932991027832031 0.895965576171875 0.851356506347656 0.799537658691406 0.740951538085938 0.676094055175781 0.605514526367188 0.529800415039062 0.449607849121094 0.365615844726562 0.278518676757812 0.189071655273438 0.0980148315429688 0.006134033203125 -0.0858001708984375 -0.177001953125 -0.266716003417969 -0.354164123535156 -0.438613891601562 -0.519355773925781 -0.595695495605469 -0.666999816894531 -0.732650756835938 -0.792106628417969 -0.844856262207031 -0.890449523925781 -0.928504943847656 -0.958702087402344 -0.980781555175781 -0.99456787109375 -0.999923706054688 -0.996818542480469 -0.985275268554688 -0.96539306640625 -0.937339782714844 -0.901351928710938 -0.85772705078125 -0.806846618652344 -0.749137878417969 -0.685081481933594 -0.615234375 -0.540168762207031 -0.460540771484375 -0.377006530761719 -0.290283203125 -0.201103210449219 -0.110221862792969 -0.0184097290039062 0.0735626220703125 0.164909362792969 0.254867553710938 0.342658996582031 0.427558898925781 0.508827209472656 0.585800170898438 0.657806396484375 0.724250793457031 0.784553527832031 0.838226318359375 0.884796142578125 0 0 0 0 0 0 0 0 0 0 0 0 0 0 0 0 0 0 0 0 0 0 0 0 0 0 0 0 0 0 0 0 0 0 0 0 0 0 0 0 0 0 0 0 0 0 0 0 0 0 0 0 0 0 0 0 0 0 0 0 0 0 0 0 0 0 0 0 0 0 0 0 0 0 0 0 0 0 0 0 0 0 0 0 0 0 0 0 0 0 0 0 0 0 0 0 0 0 0 0 0 0 0 0 0 0 0 0 0 0 0 0 0 0 0 0 0 0 0 0 0 0 0 0 0 0 0 0 0 0 0 0 0 0 0 0 0 0 0 0 0 0 0 0 0 0 0 0 0 0 0 0 0 0 0 0 0 0 0 0 0 0 0 0 0 0 0 0 0 0 0 0 0 0 0 0 0 0 0 0 0 0 0 0 0 0 0 0 0 0 0 0 0 0 0 0 0 0 0 0 0 0 0 0 0 0 0 0 0 0 0 0 0 0 0 0 0 0 0 0 0 0 0 0 0 0 0 0 0 0 0 0 0 0 0 0 0 0 0 0 0 0 0 0 0 0 0 0 0 0 0 0 0 0 0 0 0 0 0 0 0 0 0 0 0 0 0 0 0 0 0 0 0 0 0 0 0 0 0 0 0 0 0 0 0 0 0 0 0 0 0 0 0 0 0 0 0 0 0 0 0 0 0 0 0 0 0 0 0 0 0 0 0 0 0 0 0 0 0 0 0 0 0 0 0 0 0 0 0 0 0 0 0 0 0 0 0 0 0 0 0 0 0 0 0 0 0 0 0 0 0 0 0 0 0 0 0 0 0 0 0 0 0 0 0 0 0 0 0 0 0 0 0 0 0 0 0 0 0 0 0 0 0 0 0 0 0 0 0 0 0 0 0 0 0 0 0 0 0 0 0 0 0 0 0 0 0 0 0 0 0 0 0 0 0 0 0 0 0 0 0 0 0 0 0 0 0 0 0 0 0 0 0 0 0 0 0 0 0 0 0 0 0 0 0 0 0 0 0 -0.0919113159179688 -0.183036804199219 -0.272621154785156 -0.359893798828125 -0.444122314453125 -0.524589538574219 -0.600616455078125 -0.671562194824219 -0.73681640625 -0.79583740234375 -0.848121643066406 -0.893226623535156 -0.930763244628906 -0.960433959960938 -0.981964111328125 -0.995185852050781 -0.999984741210938 -0.996315002441406 -0.984207153320312 -0.963775634765625 -0.9351806640625 -0.898674011230469 -0.854560852050781 -0.803207397460938 -0.74505615234375 -0.68060302734375 -0.610382080078125 -0.534996032714844 -0.455085754394531 -0.371315002441406 -0.284408569335938 -0.195091247558594 -0.104118347167969 -0.01226806640625 0.079681396484375 0.17095947265625 0.260795593261719 0.348419189453125 0.433090209960938 0.51409912109375 0.59075927734375 0.66241455078125 0.728462219238281 0.788345336914062 0.841552734375 0.887641906738281 0.92620849609375 0.956939697265625 0.979568481445312 0.993904113769531 0.999832153320312 0.997291564941406 0.986305236816406 0.96697998046875 0.939460754394531 0.90399169921875 0.860870361328125 0.810455322265625 0.753189086914062 0.689537048339844 0.62005615234375 0.545326232910156 0.465972900390625 0 0 0 0 0 0 0 0 0 0 0 0 0 0 0 0 0 0 0 0 0 0 0 0 0 0 0 0 0 0 0 0 0 0 0 0 0 0 0 0 0 0 0 0 0 0 0 0 0 0 0 0 0 0 0 0 0 0 0 0 0 0 0 0 0 0 0 0 0 0 0 0 0 0 0 0 0 0 0 0 0 0 0 0 0 0 0 0 0 0 0 0 0 0 0 0 0 0 0 0 0 0 0 0 0 0 0 0 0 0 0 0 0 0 0 0 0 0 0 0 0 0 0 0 0 0 0 0 0 0 0 0 0 0 0 0 0 0 0 0 0 0 0 0 0 0 0 0 0 0 0 0 0 0 0 0 0 0 0 0 0 0 0 0 0 0 0 0 0 0 0 0 0 0 0 0 0 0 0 0 0 0 0 0 0 0 0 0 0 0 0 0 0 0 0 0 0 0 0 0 0 0 0 0 0 0 0 0 0 0 0 0 0 0 0 0 0 0 0 0 0 0 0 0 0 0 0 0 0 0 0 0 0 0 0 0 0 0 0 0 0 0 0 0 0 0 0 0 0 0 0 0 0 0 0 0 0 0 0 0 0 0 0 0 0 0 0 0 0 0 0 0 0 0 0 0 0 0 0 0 0 0 0 0 0 0 0 0 0 0 0 0 0 0 0 0 0 0 0 0 0 0 0 0 0 0 0 0 0 0 0 0 0 0 0 0 0 0 0 0 0 0 0 0 0 0 0 0 0 0 0 0 0 0 0 0 0 0 0 0 0 0 0 0 0 0 0 0 0 0 0 0 0 0 0 0 0 0 0 0 0 0 0 0 0 0 0 0 0 0 0 0 0 0 0 0 0 0 0 0 0 0 0 0 0 0 0 0 0 0 0 0 0 0 0 0 0 0 0 0 0 0 0 0 0 0 0 0 0 0 0 0 0 0 0 0 0 0 0 0 0 0 0 0 0 0 0 0 0 0 0 0 0 0 0 0 0 0 0 0 0 0 0 0 0 0 0 0]  distributed_mem=Block RAM  init_a=0  init_b=0  rst_a=off  rst_b=off  en_a=off  en_b=off  latency=2  write_mode_A=Read After Write  write_mode_B=Read After Write  dbl_ovrd=off  optimize=Area  use_rpm=on  block_type=dpram
  counter_b_concat : xbsIndex_r4/Concat  num_inputs=2  dbl_ovrd=off  block_type=concat
  counter_b_pad : xbsIndex_r4/Constant  const=1  gui_display_data_type=Fixed-point  arith_type=Unsigned  n_bits=1  bin_pt=0  preci_type=Single  exp_width=8  frac_width=24  explicit_period=off  period=1  equ=P=C  opselect=C  inp2=PCIN>>17  opr=+  inp1=P  carry=CIN  dbl_ovrd=off  block_type=constant
  ri_to_c : Subsystem
  w : Outport
  wires:
  Slice/1 -> cnt_sign_extb/1, cnt_sign_exta/1
  bram_din_const/1 -> coeff_mem/5, coeff_mem/2
  bram_we_const/1 -> coeff_mem/6, coeff_mem/3
  ri_to_c/1(c) -> w/1
  coeff_mem/2 -> ri_to_c/2(im)
  coeff_mem/1 -> ri_to_c/1(re)
  counter_b_concat/1 -> coeff_mem/4
  cnt_sign_exta/1 -> coeff_mem/1
  cnt_sign_extb/1 -> counter_b_concat/2
  counter_b_pad/1 -> counter_b_concat/1
  Counter/1 -> Slice/1
  rst/1 -> Counter/1

== system fft_wideband_real/fft_wideband_real/phase_mult/phase1_coeffs ==
  rst : Inport
  Counter : xbsIndex_r4/Counter  cnt_type=Free Running  cnt_to=Inf  operation=Up  start_count=0  cnt_by_val=1  arith_type=Unsigned  n_bits=6  bin_pt=0  load_pin=off  rst=on  en=off  explicit_period=on  period=1  dbl_ovrd=off  use_behavioral_HDL=off  implementation=Fabric  block_type=counter
  Slice : xbsIndex_r4/Slice  nbits=6  boolean_output=off  mode=Upper Bit Location + Width  bit1=0  base1=MSB of Input  bit0=0  base0=LSB of Input  dbl_ovrd=off  block_type=slice
  bram_din_const : xbsIndex_r4/Constant  const=0  gui_display_data_type=Fixed-point  arith_type=Signed (2's comp)  n_bits=18  bin_pt=17  preci_type=Single  exp_width=8  frac_width=24  explicit_period=off  period=1  equ=P=C  opselect=C  inp2=PCIN>>17  opr=+  inp1=P  carry=CIN  dbl_ovrd=off  block_type=constant
  bram_we_const : xbsIndex_r4/Constant  const=0  gui_display_data_type=Fixed-point  arith_type=Boolean  n_bits=16  bin_pt=14  preci_type=Single  exp_width=8  frac_width=24  explicit_period=off  period=1  equ=P=C  opselect=C  inp2=PCIN>>17  opr=+  inp1=P  carry=CIN  dbl_ovrd=off  block_type=constant
  cnt_sign_exta : xbsIndex_r4/Convert  gui_display_data_type=Fixed-point  arith_type=Unsigned  n_bits=10  bin_pt=0  float_type=Single  exp_bits=8  fraction_bits=24  quantization=Truncate  overflow=Wrap  en=off  latency=0  dbl_ovrd=off  pipeline=off  block_type=convert
  cnt_sign_extb : xbsIndex_r4/Convert  gui_display_data_type=Fixed-point  arith_type=Unsigned  n_bits=9  bin_pt=0  float_type=Single  exp_bits=8  fraction_bits=24  quantization=Truncate  overflow=Wrap  en=off  latency=0  dbl_ovrd=off  pipeline=off  block_type=convert
  coeff_mem : xbsIndex_r4/Dual Port RAM  depth=1024  initVector=[1 1 1 1 1 1 1 1 1 1 1 1 1 1 1 1 1 1 1 1 1 1 1 1 1 1 1 1 1 1 1 1 1 1 1 1 1 1 1 1 1 1 1 1 1 1 1 1 1 1 1 1 1 1 1 1 1 1 1 1 1 1 1 1 0 0 0 0 0 0 0 0 0 0 0 0 0 0 0 0 0 0 0 0 0 0 0 0 0 0 0 0 0 0 0 0 0 0 0 0 0 0 0 0 0 0 0 0 0 0 0 0 0 0 0 0 0 0 0 0 0 0 0 0 0 0 0 0 0 0 0 0 0 0 0 0 0 0 0 0 0 0 0 0 0 0 0 0 0 0 0 0 0 0 0 0 0 0 0 0 0 0 0 0 0 0 0 0 0 0 0 0 0 0 0 0 0 0 0 0 0 0 0 0 0 0 0 0 0 0 0 0 0 0 0 0 0 0 0 0 0 0 0 0 0 0 0 0 0 0 0 0 0 0 0 0 0 0 0 0 0 0 0 0 0 0 0 0 0 0 0 0 0 0 0 0 0 0 0 0 0 0 0 0 0 0 0 0 0 0 0 0 0 0 0 0 0 0 0 0 0 0 0 0 0 0 0 0 0 0 0 0 0 0 0 0 0 0 0 0 0 0 0 0 0 0 0 0 0 0 0 0 0 0 0 0 0 0 0 0 0 0 0 0 0 0 0 0 0 0 0 0 0 0 0 0 0 0 0 0 0 0 0 0 0 0 0 0 0 0 0 0 0 0 0 0 0 0 0 0 0 0 0 0 0 0 0 0 0 0 0 0 0 0 0 0 0 0 0 0 0 0 0 0 0 0 0 0 0 0 0 0 0 0 0 0 0 0 0 0 0 0 0 0 0 0 0 0 0 0 0 0 0 0 0 0 0 0 0 0 0 0 0 0 0 0 0 0 0 0 0 0 0 0 0 0 0 0 0 0 0 0 0 0 0 0 0 0 0 0 0 0 0 0 0 0 0 0 0 0 0 0 0 0 0 0 0 0 0 0 0 0 0 0 0 0 0 0 0 0 0 0 0 0 0 0 0 0 0 0 0 0 0 0 0 0 0 0 0 0 0 0 0 0 0 0 0 0 0 0 0 0 0 0 0 0 0 0 0 0 0 0 0 0 0 0 0 0 0 0 0 0 0 0 0 0 0 0 0 0 0 0 0 0 0 0 0 0 0 0 0 0 0 0 0 0 0 0 0 0 0 0 0 0 0 0 0 0 0 0 0 0 0 0 0 0 0 0 0 0 0 0 0 0 0 0 0 0 0 0 0 0 0 0 0 0 0 0 0 0 0 0 0 0 0 0 0 0 0 0 0 0 0 0 0 0 0 0 0 0 0 0 0 0 0 0 0 0 0 0 0 0 0 0 0 0 0 0 0 0 0 0 0 0 0 0 0 0 0 0 0 0 0 0 0 0 0 0 0 0 0 0 0 0 0 0 0 0 0 0 0 0 0 0 0 0 0 0 0 0 0 0 0 0 0 0 0 0 0 0 0 0 0 0 0 0 0 0 0 0 0 0 0 0 0 0 0 0 0 0 0 0 0 0 0 0 0 0 0 0 0 0 0 0 0 0 0 0 0 0 0 0 0 0 0 0 0 0 0 0 0 0 0 0 0 0 0 0 0 0 0 0 0 0 0 0 0 0 0 0 0 0 0 0 0 0 0 0 0 0 0 0 0 0 0 0 0 0 0 0 0 0 0 0 0 0 0 0 0 0 0 0 0 0 0 0 0 0 0 0 0 0 0 0 0 0 0 0 0 0 0 0 0 0 0 0 0 0 0 0 0 0 0 0 0 0 0 0 0 0 0 0 0 0 0 0 0 0 0 0 0 0 0 0 0 0 0 0 0 0 0 0 0 0 0 0 0 0 0 0 0 0 0 0 0 0 0 0 0 0 0 0 0 0 0 0 0 0 0 0 0 0 0 0 0 0 0 0 0 0 0 0 0 0 0 0 0 0 0 0 0 0 0 0 0 0 0 0 0 0 0 0 0 0 0 0 0 0 0 0 0 0 0 0 0 0 0 0 0 0 0 0 0 0 0 0 0 0 0 0 0 0 0 0 0 0 0 0 0 0 0 0 0 0 0 0 0 0 0 0 0 0 0 0 0 0 0 0 0 0 0 0 0 0 0 0 0 0 0 0 0 0 0 0 0 0 0 0 0 0 0 0 0 0 0 0 0 0 0 0 0 0 0 0 0 0 0 0 0 0 0 0 0 0 0 0 0 0 0 0 0 0 0 0 0 0 0 0 0 0 0 0 0 0 0 0 0 0 0 0 0 0 0 0]  distributed_mem=Block RAM  init_a=0  init_b=0  rst_a=off  rst_b=off  en_a=off  en_b=off  latency=2  write_mode_A=Read After Write  write_mode_B=Read After Write  dbl_ovrd=off  optimize=Area  use_rpm=on  block_type=dpram
  counter_b_concat : xbsIndex_r4/Concat  num_inputs=2  dbl_ovrd=off  block_type=concat
  counter_b_pad : xbsIndex_r4/Constant  const=1  gui_display_data_type=Fixed-point  arith_type=Unsigned  n_bits=1  bin_pt=0  preci_type=Single  exp_width=8  frac_width=24  explicit_period=off  period=1  equ=P=C  opselect=C  inp2=PCIN>>17  opr=+  inp1=P  carry=CIN  dbl_ovrd=off  block_type=constant
  ri_to_c : Subsystem
  w : Outport
  wires:
  Slice/1 -> cnt_sign_extb/1, cnt_sign_exta/1
  bram_din_const/1 -> coeff_mem/5, coeff_mem/2
  bram_we_const/1 -> coeff_mem/6, coeff_mem/3
  ri_to_c/1(c) -> w/1
  coeff_mem/2 -> ri_to_c/2(im)
  coeff_mem/1 -> ri_to_c/1(re)
  counter_b_concat/1 -> coeff_mem/4
  cnt_sign_exta/1 -> coeff_mem/1
  cnt_sign_extb/1 -> counter_b_concat/2
  counter_b_pad/1 -> counter_b_concat/1
  Counter/1 -> Slice/1
  rst/1 -> Counter/1

== system fft_wideband_real/fft_wideband_real/phase_mult/phase2_coeffs ==
  rst : Inport
  Counter : xbsIndex_r4/Counter  cnt_type=Free Running  cnt_to=Inf  operation=Up  start_count=0  cnt_by_val=1  arith_type=Unsigned  n_bits=6  bin_pt=0  load_pin=off  rst=on  en=off  explicit_period=on  period=1  dbl_ovrd=off  use_behavioral_HDL=off  implementation=Fabric  block_type=counter
  Slice : xbsIndex_r4/Slice  nbits=6  boolean_output=off  mode=Upper Bit Location + Width  bit1=0  base1=MSB of Input  bit0=0  base0=LSB of Input  dbl_ovrd=off  block_type=slice
  bram_din_const : xbsIndex_r4/Constant  const=0  gui_display_data_type=Fixed-point  arith_type=Signed (2's comp)  n_bits=18  bin_pt=17  preci_type=Single  exp_width=8  frac_width=24  explicit_period=off  period=1  equ=P=C  opselect=C  inp2=PCIN>>17  opr=+  inp1=P  carry=CIN  dbl_ovrd=off  block_type=constant
  bram_we_const : xbsIndex_r4/Constant  const=0  gui_display_data_type=Fixed-point  arith_type=Boolean  n_bits=16  bin_pt=14  preci_type=Single  exp_width=8  frac_width=24  explicit_period=off  period=1  equ=P=C  opselect=C  inp2=PCIN>>17  opr=+  inp1=P  carry=CIN  dbl_ovrd=off  block_type=constant
  cnt_sign_exta : xbsIndex_r4/Convert  gui_display_data_type=Fixed-point  arith_type=Unsigned  n_bits=10  bin_pt=0  float_type=Single  exp_bits=8  fraction_bits=24  quantization=Truncate  overflow=Wrap  en=off  latency=0  dbl_ovrd=off  pipeline=off  block_type=convert
  cnt_sign_extb : xbsIndex_r4/Convert  gui_display_data_type=Fixed-point  arith_type=Unsigned  n_bits=9  bin_pt=0  float_type=Single  exp_bits=8  fraction_bits=24  quantization=Truncate  overflow=Wrap  en=off  latency=0  dbl_ovrd=off  pipeline=off  block_type=convert
  coeff_mem : xbsIndex_r4/Dual Port RAM  depth=1024  initVector=[1 0.999984741210938 0.999923706054688 0.999832153320312 0.999702453613281 0.999526977539062 0.999320983886719 0.999076843261719 0.998794555664062 0.99847412109375 0.998115539550781 0.997726440429688 0.997291564941406 0.996818542480469 0.996315002441406 0.995765686035156 0.995185852050781 0.99456787109375 0.993904113769531 0.993209838867188 0.992477416992188 0.991706848144531 0.99090576171875 0.990058898925781 0.989173889160156 0.988258361816406 0.9873046875 0.986305236816406 0.985275268554688 0.984207153320312 0.983108520507812 0.981964111328125 0.980781555175781 0.979568481445312 0.978317260742188 0.977027893066406 0.975700378417969 0.974342346191406 0.972938537597656 0.971504211425781 0.97003173828125 0.968521118164062 0.96697998046875 0.96539306640625 0.963775634765625 0.962120056152344 0.960433959960938 0.958702087402344 0.956939697265625 0.95513916015625 0.95330810546875 0.951431274414062 0.949531555175781 0.947586059570312 0.945610046386719 0.943595886230469 0.941543579101562 0.939460754394531 0.937339782714844 0.9351806640625 0.932991027832031 0.930763244628906 0.928504943847656 0.92620849609375 0 0 0 0 0 0 0 0 0 0 0 0 0 0 0 0 0 0 0 0 0 0 0 0 0 0 0 0 0 0 0 0 0 0 0 0 0 0 0 0 0 0 0 0 0 0 0 0 0 0 0 0 0 0 0 0 0 0 0 0 0 0 0 0 0 0 0 0 0 0 0 0 0 0 0 0 0 0 0 0 0 0 0 0 0 0 0 0 0 0 0 0 0 0 0 0 0 0 0 0 0 0 0 0 0 0 0 0 0 0 0 0 0 0 0 0 0 0 0 0 0 0 0 0 0 0 0 0 0 0 0 0 0 0 0 0 0 0 0 0 0 0 0 0 0 0 0 0 0 0 0 0 0 0 0 0 0 0 0 0 0 0 0 0 0 0 0 0 0 0 0 0 0 0 0 0 0 0 0 0 0 0 0 0 0 0 0 0 0 0 0 0 0 0 0 0 0 0 0 0 0 0 0 0 0 0 0 0 0 0 0 0 0 0 0 0 0 0 0 0 0 0 0 0 0 0 0 0 0 0 0 0 0 0 0 0 0 0 0 0 0 0 0 0 0 0 0 0 0 0 0 0 0 0 0 0 0 0 0 0 0 0 0 0 0 0 0 0 0 0 0 0 0 0 0 0 0 0 0 0 0 0 0 0 0 0 0 0 0 0 0 0 0 0 0 0 0 0 0 0 0 0 0 0 0 0 0 0 0 0 0 0 0 0 0 0 0 0 0 0 0 0 0 0 0 0 0 0 0 0 0 0 0 0 0 0 0 0 0 0 0 0 0 0 0 0 0 0 0 0 0 0 0 0 0 0 0 0 0 0 0 0 0 0 0 0 0 0 0 0 0 0 0 0 0 0 0 0 0 0 0 0 0 0 0 0 0 0 0 0 0 0 0 0 0 0 0 0 0 0 0 0 0 0 0 0 0 0 0 0 0 0 0 0 0 0 0 0 0 0 0 0 0 0 0 0 0 0 0 0 0 0 0 0 0 0 0 0 0 0 0 0 0 0 0 0 0 0 0 -0.006134033203125 -0.01226806640625 -0.0184097290039062 -0.0245437622070312 -0.0306777954101562 -0.03680419921875 -0.042938232421875 -0.0490646362304688 -0.0551986694335938 -0.0613174438476562 -0.06744384765625 -0.0735626220703125 -0.079681396484375 -0.0858001708984375 -0.0919113159179688 -0.0980148315429688 -0.104118347167969 -0.110221862792969 -0.116317749023438 -0.122413635253906 -0.128501892089844 -0.13458251953125 -0.140655517578125 -0.146728515625 -0.152793884277344 -0.158859252929688 -0.164909362792969 -0.17095947265625 -0.177001953125 -0.183036804199219 -0.189071655273438 -0.195091247558594 -0.201103210449219 -0.207115173339844 -0.213111877441406 -0.219100952148438 -0.225082397460938 -0.231056213378906 -0.237022399902344 -0.24298095703125 -0.248924255371094 -0.254867553710938 -0.260795593261719 -0.266716003417969 -0.272621154785156 -0.278518676757812 -0.284408569335938 -0.290283203125 -0.296150207519531 -0.302009582519531 -0.307846069335938 -0.313682556152344 -0.319503784179688 -0.325309753417969 -0.331108093261719 -0.336891174316406 -0.342658996582031 -0.348419189453125 -0.354164123535156 -0.359893798828125 -0.365615844726562 -0.371315002441406 -0.377006530761719 0 0 0 0 0 0 0 0 0 0 0 0 0 0 0 0 0 0 0 0 0 0 0 0 0 0 0 0 0 0 0 0 0 0 0 0 0 0 0 0 0 0 0 0 0 0 0 0 0 0 0 0 0 0 0 0 0 0 0 0 0 0 0 0 0 0 0 0 0 0 0 0 0 0 0 0 0 0 0 0 0 0 0 0 0 0 0 0 0 0 0 0 0 0 0 0 0 0 0 0 0 0 0 0 0 0 0 0 0 0 0 0 0 0 0 0 0 0 0 0 0 0 0 0 0 0 0 0 0 0 0 0 0 0 0 0 0 0 0 0 0 0 0 0 0 0 0 0 0 0 0 0 0 0 0 0 0 0 0 0 0 0 0 0 0 0 0 0 0 0 0 0 0 0 0 0 0 0 0 0 0 0 0 0 0 0 0 0 0 0 0 0 0 0 0 0 0 0 0 0 0 0 0 0 0 0 0 0 0 0 0 0 0 0 0 0 0 0 0 0 0 0 0 0 0 0 0 0 0 0 0 0 0 0 0 0 0 0 0 0 0 0 0 0 0 0 0 0 0 0 0 0 0 0 0 0 0 0 0 0 0 0 0 0 0 0 0 0 0 0 0 0 0 0 0 0 0 0 0 0 0 0 0 0 0 0 0 0 0 0 0 0 0 0 0 0 0 0 0 0 0 0 0 0 0 0 0 0 0 0 0 0 0 0 0 0 0 0 0 0 0 0 0 0 0 0 0 0 0 0 0 0 0 0 0 0 0 0 0 0 0 0 0 0 0 0 0 0 0 0 0 0 0 0 0 0 0 0 0 0 0 0 0 0 0 0 0 0 0 0 0 0 0 0 0 0 0 0 0 0 0 0 0 0 0 0 0 0 0 0 0 0 0 0 0 0 0 0 0 0 0 0 0 0 0 0 0 0 0 0 0 0 0 0 0 0 0 0 0 0 0 0 0 0 0 0 0 0 0 0 0 0 0 0 0 0 0 0 0 0 0 0 0 0 0 0 0 0]  distributed_mem=Block RAM  init_a=0  init_b=0  rst_a=off  rst_b=off  en_a=off  en_b=off  latency=2  write_mode_A=Read After Write  write_mode_B=Read After Write  dbl_ovrd=off  optimize=Area  use_rpm=on  block_type=dpram
  counter_b_concat : xbsIndex_r4/Concat  num_inputs=2  dbl_ovrd=off  block_type=concat
  counter_b_pad : xbsIndex_r4/Constant  const=1  gui_display_data_type=Fixed-point  arith_type=Unsigned  n_bits=1  bin_pt=0  preci_type=Single  exp_width=8  frac_width=24  explicit_period=off  period=1  equ=P=C  opselect=C  inp2=PCIN>>17  opr=+  inp1=P  carry=CIN  dbl_ovrd=off  block_type=constant
  ri_to_c : Subsystem
  w : Outport
  wires:
  Slice/1 -> cnt_sign_extb/1, cnt_sign_exta/1
  bram_din_const/1 -> coeff_mem/5, coeff_mem/2
  bram_we_const/1 -> coeff_mem/6, coeff_mem/3
  ri_to_c/1(c) -> w/1
  coeff_mem/2 -> ri_to_c/2(im)
  coeff_mem/1 -> ri_to_c/1(re)
  counter_b_concat/1 -> coeff_mem/4
  cnt_sign_exta/1 -> coeff_mem/1
  cnt_sign_extb/1 -> counter_b_concat/2
  counter_b_pad/1 -> counter_b_concat/1
  Counter/1 -> Slice/1
  rst/1 -> Counter/1
